simulink subsystem "Read_Arm"  (R2024a)
settings: Solver=VariableStepAuto  StartTime=0.0  StopTime=10.0  RelTol=1e-3
settings Model: Creator=gurt1  LastModifiedBy=gurt1

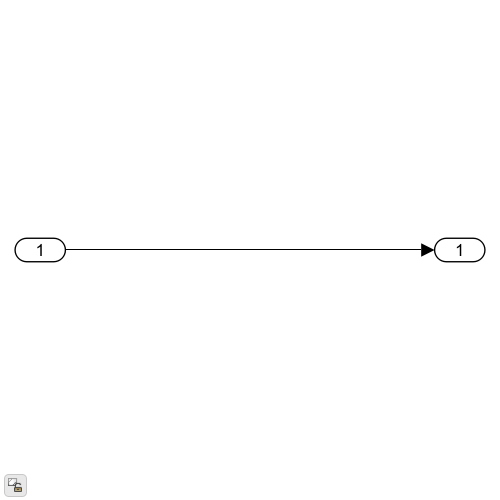
[thumbnail: Simulink's stored preview of the top-level diagram]
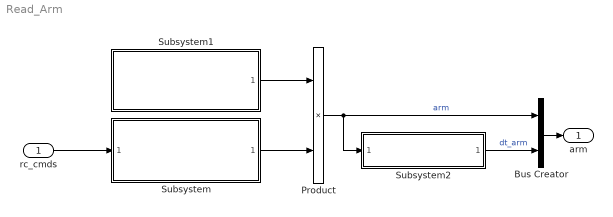
== system Read_Arm ==
  rc_cmds : Inport
  Bus Creator : BusCreator  Inputs=2
  Product : Product
  Subsystem : Subsystem  ReferencedSubsystem=Pilot_arm
  Subsystem1 : Subsystem  ReferencedSubsystem=PX4_arm
  Subsystem2 : Subsystem  ReferencedSubsystem=arm_time
  arm : Outport
  wires:
  Product/1 -> Subsystem2/1, Bus Creator/1  "arm"
  rc_cmds/1 -> Subsystem/1
  Subsystem/1 -> Product/2
  Subsystem1/1 -> Product/1
  Bus Creator/1 -> arm/1
  Subsystem2/1 -> Bus Creator/2  "dt_arm"
